simulink model "HW4"  (R2015b)
settings: Solver=VariableStepAuto  StartTime=0.0  StopTime=37.5  RelTol=1e-3
libraries: simulink x9
settings Model: Creator=YagfarovRauf  LastModifiedBy=YagfarovRauf

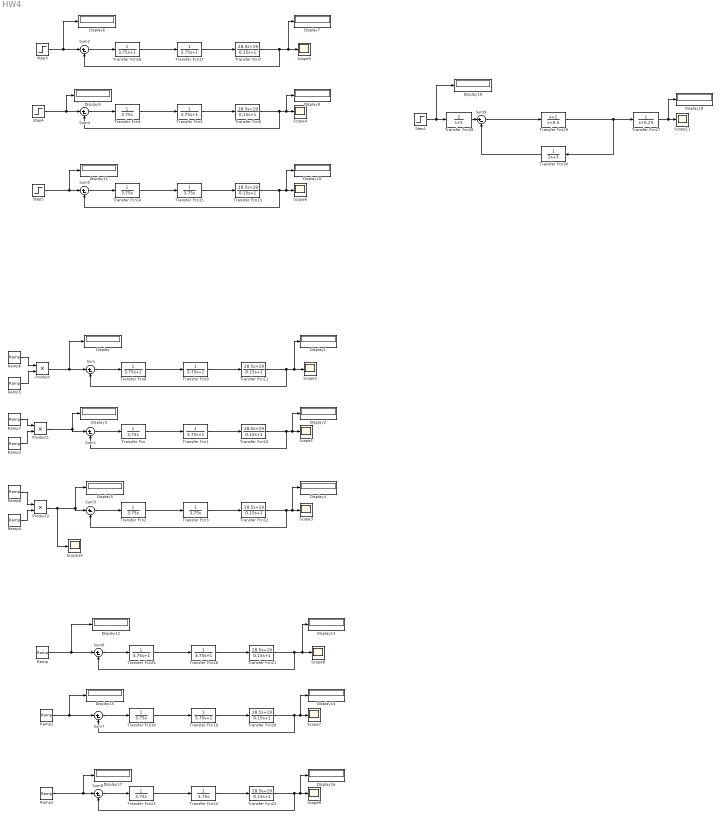
== system HW4 ==
  Display{,1..19} (20 alike) : Display
  Product : Product
  Product1 : Product
  Product2 : Product
  Ramp{,1..8} (9 alike) : simulink/Sources/Ramp  slope=1  start=0  X0=0
  Scope{1..11} (11 alike) : Scope
  Step{1,3..5} (4 alike) : Step  SampleTime=0
  Sum{,1..9} (10 alike) : Sum  Inputs=|+-
  Transfer Fcn{,2..4,14..15,18,23..24} (9 alike) : TransferFcn  Denominator=[3.75 0]
  Transfer Fcn{1,5,8..9,16..17,19,25..26} (9 alike) : TransferFcn  Denominator=[3.75 1]
  Transfer Fcn{6..7,10..13,20..22} (9 alike) : TransferFcn  Numerator=[28.5 19]  Denominator=[0.15 1]
  Transfer Fcn27 : TransferFcn  Denominator=[1 0.25]
  Transfer Fcn28 : TransferFcn  Numerator=[2]  Denominator=[1 5]
  Transfer Fcn29 : TransferFcn  Numerator=[1 1]  Denominator=[1 0.5]
  Transfer Fcn30 : TransferFcn  Denominator=[2 3]
  wires:
  Transfer Fcn/1 -> Transfer Fcn1/1
  Transfer Fcn1/1 -> Transfer Fcn10/1
  Transfer Fcn8/1 -> Transfer Fcn9/1
  Transfer Fcn9/1 -> Transfer Fcn11/1
  Sum/1 -> Transfer Fcn8/1
  Sum1/1 -> Transfer Fcn/1
  Transfer Fcn11/1 -> Display1/1, Scope2/1, Sum/2
  Transfer Fcn10/1 -> Display2/1, Scope1/1, Sum1/2
  Transfer Fcn2/1 -> Transfer Fcn3/1
  Transfer Fcn3/1 -> Transfer Fcn12/1
  Sum3/1 -> Transfer Fcn2/1
  Transfer Fcn12/1 -> Display4/1, Scope3/1, Sum3/2
  Transfer Fcn4/1 -> Transfer Fcn5/1
  Transfer Fcn5/1 -> Transfer Fcn6/1
  Transfer Fcn16/1 -> Transfer Fcn17/1
  Transfer Fcn17/1 -> Transfer Fcn7/1
  Sum2/1 -> Transfer Fcn16/1
  Sum4/1 -> Transfer Fcn4/1
  Transfer Fcn7/1 -> Display7/1, Scope5/1, Sum2/2
  Transfer Fcn6/1 -> Display8/1, Scope4/1, Sum4/2
  Transfer Fcn14/1 -> Transfer Fcn15/1
  Transfer Fcn15/1 -> Transfer Fcn13/1
  Sum5/1 -> Transfer Fcn14/1
  Transfer Fcn13/1 -> Display10/1, Scope6/1, Sum5/2
  Step4/1 -> Display9/1, Sum4/1
  Step5/1 -> Display11/1, Sum5/1
  Step3/1 -> Display6/1, Sum2/1
  Transfer Fcn18/1 -> Transfer Fcn19/1
  Transfer Fcn19/1 -> Transfer Fcn20/1
  Transfer Fcn25/1 -> Transfer Fcn26/1
  Transfer Fcn26/1 -> Transfer Fcn21/1
  Sum6/1 -> Transfer Fcn25/1
  Sum7/1 -> Transfer Fcn18/1
  Transfer Fcn21/1 -> Display13/1, Scope8/1, Sum6/2
  Transfer Fcn20/1 -> Display14/1, Scope7/1, Sum7/2
  Transfer Fcn23/1 -> Transfer Fcn24/1
  Transfer Fcn24/1 -> Transfer Fcn22/1
  Sum8/1 -> Transfer Fcn23/1
  Transfer Fcn22/1 -> Display16/1, Scope9/1, Sum8/2
  Product/1 -> Display/1, Sum/1
  Product1/1 -> Sum1/1, Display3/1
  Product2/1 -> Scope10/1, Sum3/1, Display5/1
  Ramp/1 -> Display12/1, Sum6/1
  Ramp1/1 -> Display15/1, Sum7/1
  Ramp2/1 -> Display17/1, Sum8/1
  Ramp6/1 -> Product/1
  Ramp5/1 -> Product/2
  Ramp7/1 -> Product1/1
  Ramp3/1 -> Product1/2
  Ramp4/1 -> Product2/2
  Ramp8/1 -> Product2/1
  Sum9/1 -> Transfer Fcn29/1
  Transfer Fcn29/1 -> Transfer Fcn30/1, Transfer Fcn27/1
  Step1/1 -> Display19/1, Transfer Fcn28/1
  Transfer Fcn28/1 -> Sum9/1
  Transfer Fcn27/1 -> Display18/1, Scope11/1
  Transfer Fcn30/1 -> Sum9/2
